simulink model "Three_Phase_Rectifier_HalfControlled_Rload_90deg"  (R2018b)
settings: Solver=VariableStepAuto  StartTime=0.0  StopTime=0.06  RelTol=1e-3
libraries: powerlib x24
settings Model: Creator=A.hey  LastModifiedBy=A.hey

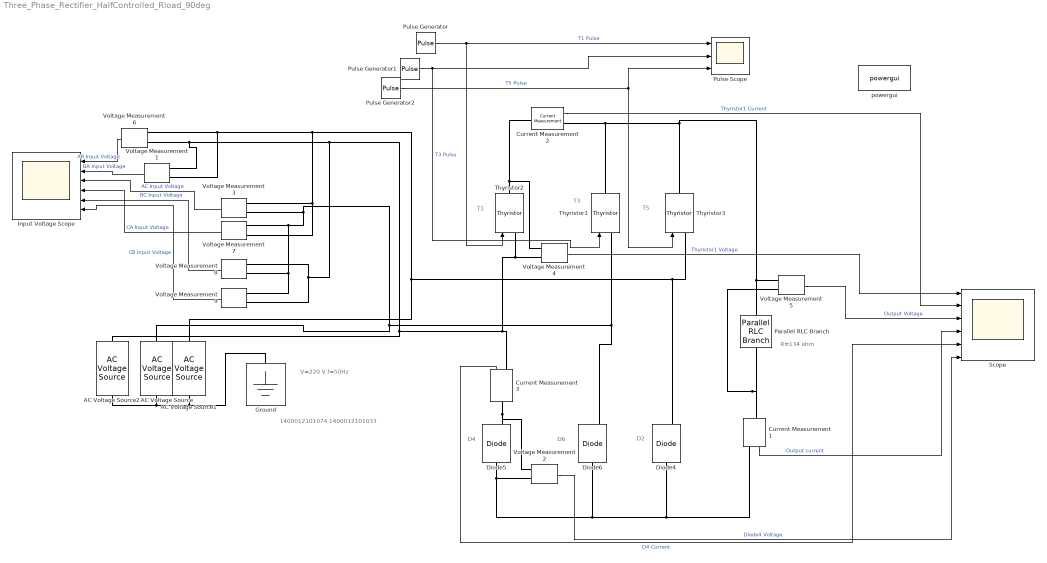
== system Three_Phase_Rectifier_HalfControlled_Rload_90deg ==
  note: T5
  note: D2
  note: 1400012101074
      | 1400012101033
  note: D4
  note: D6
  note: V=220 V
      | f=50Hz
  note: R=134 ohm
  note: T1
  note: T3
  " Scope " : Scope  NumInputPorts=6
  AC Voltage Source : powerlib/Electrical Sources/AC Voltage Source  Amplitude=220  Phase=-120  Frequency=50  SampleTime=0  Measurements=None  BusType=swing  Pref=10e3  Qref=0  Qmin=-inf  Qmax=+inf
  AC Voltage Source1 : powerlib/Electrical Sources/AC Voltage Source  Amplitude=220  Phase=-240  Frequency=50  SampleTime=0  Measurements=None  BusType=swing  Pref=10e3  Qref=0  Qmin=-inf  Qmax=+inf
  AC Voltage Source2 : powerlib/Electrical Sources/AC Voltage Source  Amplitude=220  Phase=0  Frequency=50  SampleTime=0  Measurements=None  BusType=swing  Pref=10e3  Qref=0  Qmin=-inf  Qmax=+inf
  Current Measurement1 : powerlib/Measurements/Current Measurement  PhasorSimulation=off  OutputType=Complex  PSBequivalent=0
  Current Measurement2 : powerlib/Measurements/Current Measurement  PhasorSimulation=off  OutputType=Complex  PSBequivalent=0
  Current Measurement3 : powerlib/Measurements/Current Measurement  PhasorSimulation=off  OutputType=Complex  PSBequivalent=0
  Diode4 : powerlib/Power Electronics/Diode  Ron=0.001  Lon=0  Vf=0.8  IC=0  UseSnubber=0  Rs=500  Cs=250e-9  Measurements=on
  Diode5 : powerlib/Power Electronics/Diode  Ron=0.001  Lon=0  Vf=0.8  IC=0  UseSnubber=0  Rs=500  Cs=250e-9  Measurements=on
  Diode6 : powerlib/Power Electronics/Diode  Ron=0.001  Lon=0  Vf=0.8  IC=0  UseSnubber=0  Rs=500  Cs=250e-9  Measurements=on
  Ground : powerlib/Elements/Ground  LConnTagsString=a
  "Input Voltage Scope " : Scope  NumInputPorts=6
  Parallel RLC Branch : powerlib/Elements/Parallel RLC Branch  LConnTagsString=a  RConnTagsString=__new0  BranchType=R  Resistance=134  Inductance=1e-3  SetiL0=off  InitialCurrent=0  Capacitance=1e-6  Setx0=off  InitialVoltage=0  Measurements=None
  Pulse Generator : DiscretePulseGenerator  PulseType=Time based  Amplitude=10  Period=0.02  PulseWidth=50  PhaseDelay=(0.01/6)+(0.01/2)
  Pulse Generator1 : DiscretePulseGenerator  PulseType=Time based  Amplitude=10  Period=0.02  PulseWidth=50  PhaseDelay=(0.05/6 )+(0.01/2)
  Pulse Generator2 : DiscretePulseGenerator  PulseType=Time based  Amplitude=10  Period=0.02  PulseWidth=50  PhaseDelay=(0.09/6)+(0.01/2)
  Pulse Scope : Scope  NumInputPorts=3
  Thyristor1 : powerlib/Power Electronics/Thyristor  Ron=0.001  Lon=0  Vf=0.1  IC=0  Rs=500  Cs=250e-9  Measurements=off
      settings: SourceProductName=Simscape Electrical
  Thyristor2 : powerlib/Power Electronics/Thyristor  Ron=0.001  Lon=0  Vf=0.1  IC=0  Rs=500  Cs=250e-9  Measurements=off
      settings: SourceProductName=Simscape Electrical
  Thyristor3 : powerlib/Power Electronics/Thyristor  Ron=0.001  Lon=0  Vf=0.1  IC=0  Rs=500  Cs=250e-9  Measurements=off
      settings: SourceProductName=Simscape Electrical
  Voltage Measurement{1..9} (9 alike) : powerlib/Measurements/Voltage Measurement  PhasorSimulation=off  OutputType=Complex  PSBequivalent=0
  powergui : powerlib/powergui  Priority=1  SimulationMode=Continuous  SampleTime=50e-6  frequency=60  Iterations=50  frequencyindice=50  Pbase=100e6  ErrMax=1e-4  UnitsV=kV  UnitsW=MW  buscounter=0  FunctionMessages=off  echomessages=off  EnableUseOfTLC=off  CurrentSourceSwitches=off  DisableSnubberDevices=off  DisableRonSwitches=off  DisableVfSwitches=off  DisplayEquations=off  SolverType=Tustin/Backward Euler (TBE)  Interpol=off  ExternalGateDelay=off  methode=off  Ts=100  x0status=blocks  SPID=on  SwTol=0  HookPort=off  RestoreLinks=warning  ResistiveCurrentMeasurement=off  Frange=[0:2:500]  Ylog=off  Xlog=on  ShowGrid=off  save=off  variable=ZData  structure=0  ZoomFFT=off  StartTime=0.0  cycles=1  DisplayStyle=1  fundamental=60  FreqAxis=off  MaxFrequency=1000  frequencyindicesteady=1  RmsSteady=1  display=off
  wires:
  Voltage Measurement1/1 -> "Input Voltage Scope "/2  "BA Input Voltage"
  Current Measurement2/1 -> " Scope "/2  "Thyristor1 Current"
  Voltage Measurement4/1 -> " Scope "/1  "Thyristor1 Voltage"
  Current Measurement1/1 -> " Scope "/4  "Output current"
  Voltage Measurement6/1 -> "Input Voltage Scope "/1  "AB Input Voltage"
  Voltage Measurement7/1 -> "Input Voltage Scope "/4  "CA Input Voltage"
  Voltage Measurement3/1 -> "Input Voltage Scope "/3  "AC Input Voltage"
  Voltage Measurement8/1 -> "Input Voltage Scope "/5  "BC Input Voltage"
  Voltage Measurement9/1 -> "Input Voltage Scope "/6  "CB Input Voltage"
  Voltage Measurement5/1 -> " Scope "/3  "Output Voltage"
  Pulse Generator/1 -> Thyristor2/1, Pulse Scope/1  "T1 Pulse"
  Pulse Generator1/1 -> Pulse Scope/2, Thyristor1/1  "T3 Pulse"
  Pulse Generator2/1 -> Pulse Scope/3, Thyristor3/1  "T5 Pulse"
  Current Measurement3/1 -> " Scope "/5  "D4 Current"
  Voltage Measurement2/1 -> " Scope "/6  "Diode4 Voltage"
  connections:
  Voltage Measurement3/LConn1 -- AC Voltage Source1/RConn1 -- Thyristor3/LConn1 -- Diode4/RConn1 -- Voltage Measurement6/LConn1 -- Voltage Measurement1/LConn2 -- Voltage Measurement7/LConn2
  Voltage Measurement4/LConn2 -- Thyristor2/RConn1 -- Current Measurement2/LConn1
  Current Measurement1/LConn1 -- Voltage Measurement5/LConn2 -- Parallel RLC Branch/RConn1
  Voltage Measurement6/LConn2 -- AC Voltage Source2/RConn1 -- Current Measurement3/RConn1 -- Thyristor2/LConn1 -- Voltage Measurement4/LConn1 -- Voltage Measurement8/LConn1 -- Voltage Measurement9/LConn2 -- Voltage Measurement1/LConn1
  Voltage Measurement5/LConn1 -- Parallel RLC Branch/LConn1 -- Thyristor3/RConn1 -- Current Measurement2/RConn1 -- Thyristor1/RConn1
  Diode5/LConn1 -- Voltage Measurement2/LConn1 -- Diode4/LConn1 -- Current Measurement1/RConn1 -- Diode6/LConn1
  AC Voltage Source1/LConn1 -- AC Voltage Source2/LConn1 -- AC Voltage Source/LConn1 -- Ground/LConn1
  Voltage Measurement8/LConn2 -- Voltage Measurement9/LConn1 -- Voltage Measurement7/LConn1 -- AC Voltage Source/RConn1 -- Thyristor1/LConn1 -- Diode6/RConn1 -- Voltage Measurement3/LConn2
  Diode5/RConn1 -- Current Measurement3/LConn1 -- Voltage Measurement2/LConn2
